simulink model "hw"  (R2021a)
settings: Solver=VariableStepAuto  StartTime=0.0  StopTime=10  RelTol=1e-3
settings Model: Creator=Wasif  LastModifiedBy=Wasif

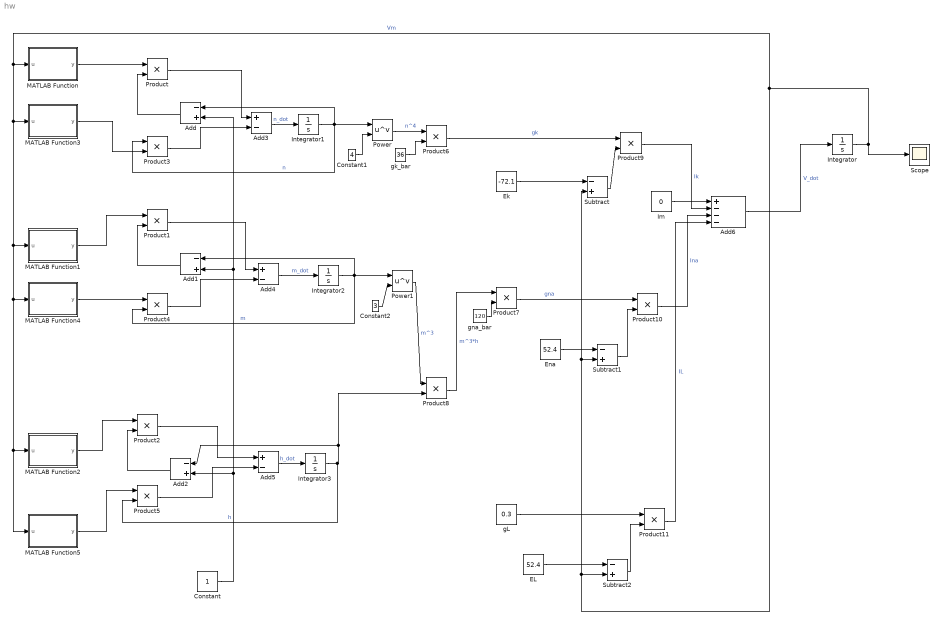
== system hw ==
  Add : Sum  Inputs=-+
  Add1 : Sum  Inputs=-+
  Add2 : Sum  Inputs=-+
  Add3 : Sum  Inputs=+-
  Add4 : Sum  Inputs=+-
  Add5 : Sum  Inputs=+-
  Add6 : Sum  Inputs=+---
  Constant : Constant
  Constant1 : Constant  Value=4
  Constant2 : Constant  Value=3
  EL : Constant  Value=52.4
  Ek : Constant  Value=-72.1
  Ena : Constant  Value=52.4
  Im : Constant  Value=0
  Integrator : Integrator
  Integrator1 : Integrator  InitialCondition=0.378
  Integrator2 : Integrator  InitialCondition=0.417
  Integrator3 : Integrator  InitialCondition=0.477
  MATLAB Function : MATLAB Function  TreatAsAtomicUnit=on
  MATLAB Function1 : MATLAB Function  TreatAsAtomicUnit=on
  MATLAB Function2 : MATLAB Function  TreatAsAtomicUnit=on
  MATLAB Function3 : MATLAB Function  TreatAsAtomicUnit=on
  MATLAB Function4 : MATLAB Function  TreatAsAtomicUnit=on
  MATLAB Function5 : MATLAB Function  TreatAsAtomicUnit=on
  Power : Math  Operator=pow  SaturateOnIntegerOverflow=on
  Power1 : Math  Operator=pow  SaturateOnIntegerOverflow=on
  Product{,1..11} (12 alike) : Product
  Scope : Scope
  Subtract : Sum  Inputs=-+
  Subtract1 : Sum  Inputs=-+
  Subtract2 : Sum  Inputs=-+
  gL : Constant  Value=0.3
  gk_bar : Constant  Value=36
  gna_bar : Constant  Value=120
  wires:
  Add6/1 -> Integrator/1  "V_dot"
  Integrator1/1 -> Power/1, Add/1, Product3/1  "n"
  Add3/1 -> Integrator1/1  "n_dot"
  Add4/1 -> Integrator2/1  "m_dot"
  Integrator3/1 -> Product5/2, Product8/2, Add2/1  "h"
  Add5/1 -> Integrator3/1  "h_dot"
  Constant/1 -> Add2/2, Add1/2, Add/2
  Add/1 -> Product/2
  Add1/1 -> Product1/2
  Add2/1 -> Product2/2
  MATLAB Function/1(y) -> Product/1
  MATLAB Function3/1(y) -> Product3/2
  Product3/1 -> Add3/2
  Product/1 -> Add3/1
  MATLAB Function1/1(y) -> Product1/1
  MATLAB Function4/1(y) -> Product4/1
  Product1/1 -> Add4/1
  Product4/1 -> Add4/2
  MATLAB Function2/1(y) -> Product2/1
  MATLAB Function5/1(y) -> Product5/1
  Product5/1 -> Add5/2
  Product2/1 -> Add5/1
  Constant1/1 -> Power/2
  Power/1 -> Product6/1  "n^4"
  gk_bar/1 -> Product6/2
  Product6/1 -> Product9/1  "gk"
  Product8/1 -> Product7/1  "m^3*h"
  Product7/1 -> Product10/1  "gna"
  gna_bar/1 -> Product7/2
  Integrator2/1 -> Power1/1, Add1/1, Product4/2  "m"
  Constant2/1 -> Power1/2
  Power1/1 -> Product8/1  "m^3"
  Subtract/1 -> Product9/2
  Subtract1/1 -> Product10/2
  Ek/1 -> Subtract/1
  Ena/1 -> Subtract1/1
  Integrator/1 -> Scope/1, MATLAB Function1/1(u), MATLAB Function4/1(u), MATLAB Function5/1(u), MATLAB Function2/1(u), MATLAB Function3/1(u), MATLAB Function/1(u), Subtract2/2, Subtract/2, Subtract1/2  "Vm"
  EL/1 -> Subtract2/1
  Subtract2/1 -> Product11/2
  gL/1 -> Product11/1
  Product9/1 -> Add6/2  "Ik"
  Product10/1 -> Add6/3  "Ina"
  Product11/1 -> Add6/4  "IL"
  Im/1 -> Add6/1

== matlab function hw/MATLAB Function ==
  data: u input; y output
function y = alphan(u)
vm=u+60
alpha_m=(0.01*(10-vm))/(exp((10-vm)/10)-1)

y = alpha_m;

== matlab function hw/MATLAB Function2 ==
  data: u input; y output
function y = alphah(u)
vm=u+60;
alpha_h=0.07*exp(-vm/20)

y = alpha_h;

== matlab function hw/MATLAB Function3 ==
  data: u input; y output
function y = betan(u)
vm=u+60;
beta_n=0.125*exp(-vm/80)

y = beta_n;

== matlab function hw/MATLAB Function4 ==
  data: u input; y output
function y = betam(u)
vm=u+60;
beta_m=4*exp(-vm/18)

y = beta_m;

== matlab function hw/MATLAB Function5 ==
  data: u input; y output
function y = betah(u)
vm=u+60;
beta_h=1/(exp((30-vm)/10)+1)

y = beta_h;

== matlab function hw/MATLAB Function1 ==
  data: u input; y output
function y = alpham(u)
vm=u+60
alpha_n=(0.1*(25-vm))/(exp((25-vm)/10)-1)

y = alpha_n;
